simulink model "lab4_prep"  (R2023b)
settings: Solver=VariableStepAuto  StartTime=0.0  StopTime=10.0  RelTol=10e-10  AbsTol=10e-10
values from neighbouring files (symbols this model uses):
  Actrl = A + B*K - L*C    [lab4.m]
  Bctrl = [L, -B*K]    [lab4.m]
  C = [1 0 0 0; 0 0 1 0]    [lab4.m]
  Cctrl = K    [lab4.m]
  Dctrl = [zeros(1,2), -K]    [lab4.m]
  K = -place(A,B,p_K)    [lab4.m]
  Ulim = 5.875    [lab4.m]
  x0 = [0; 0; pi/24; 0]    [lab4.m]
settings Model: Creator=Darrian  LastModifiedBy=Darrian

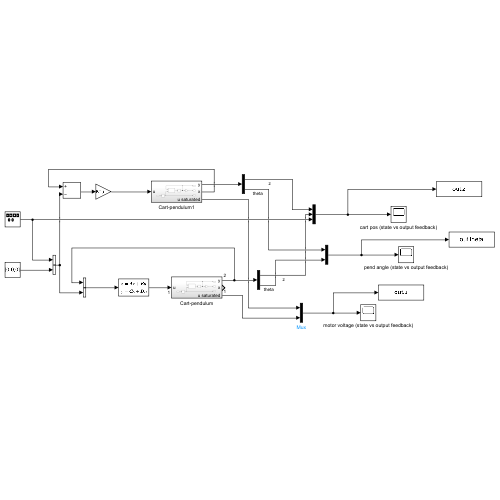
[thumbnail: Simulink's stored preview of the top-level diagram]
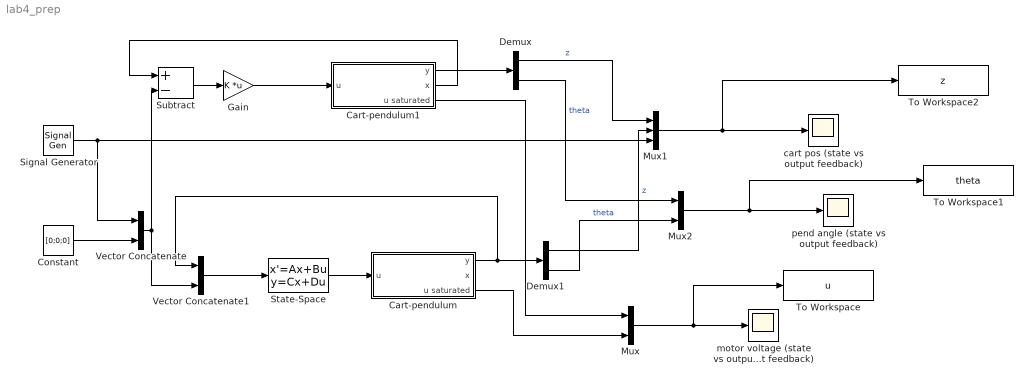
== system lab4_prep ==
  Cart-pendulum : Subsystem
  Cart-pendulum1 : Subsystem
  Constant : Constant  Value=[0;0;0]
  Demux : Demux  Outputs=2
  Demux1 : Demux  Outputs=2
  Gain : Gain  Gain=K  Multiplication=Matrix(K*u)
  Mux : Mux  Inputs=2
  Mux1 : Mux  Inputs=3
  Mux2 : Mux  Inputs=2
  Signal Generator : SignalGenerator  WaveForm=square  Amplitude=0.1  Frequency=0.1
  State-Space : StateSpace  A=Actrl  B=Bctrl  C=Cctrl  D=Dctrl  InitialCondition=0
  Subtract : Sum  Inputs=+-
  To Workspace : ToWorkspace  VariableName=u  SaveFormat=Timeseries  SampleTime=-1
  To Workspace1 : ToWorkspace  VariableName=theta  SaveFormat=Timeseries  SampleTime=-1
  To Workspace2 : ToWorkspace  VariableName=z  SaveFormat=Timeseries  SampleTime=-1
  Vector Concatenate : Concatenate
  Vector Concatenate1 : Concatenate
  cart pos (state vs output feedback) : Scope
  motor voltage (state vs output feedback) : Scope
  pend angle (state vs output feedback) : Scope
  wires:
  Gain/1 -> Cart-pendulum1/1(u)
  Constant/1 -> Vector Concatenate/2
  Signal Generator/1 -> Mux1/3, Vector Concatenate/1
  Subtract/1 -> Gain/1
  Cart-pendulum1/2(x) -> Subtract/1
  Cart-pendulum1/1(y) -> Demux/1
  State-Space/1 -> Cart-pendulum/1(u)
  Vector Concatenate/1 -> Subtract/2, Vector Concatenate1/2
  Vector Concatenate1/1 -> State-Space/1
  Cart-pendulum/1(y) -> Vector Concatenate1/1, Demux1/1
  Cart-pendulum1/3(u saturated) -> Mux/1
  Cart-pendulum/3(u saturated) -> Mux/2
  Demux/2 -> Mux2/1  "theta"
  Demux1/2 -> Mux2/2  "theta"
  Demux1/1 -> Mux1/2  "z"
  Demux/1 -> Mux1/1  "z"
  Mux/1 -> To Workspace/1, motor voltage (state vs output feedback)/1
  Mux1/1 -> To Workspace2/1, cart pos (state vs output feedback)/1
  Mux2/1 -> To Workspace1/1, pend angle (state vs output feedback)/1

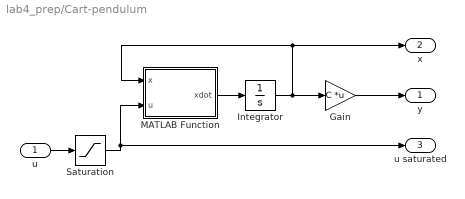
== system lab4_prep/Cart-pendulum ==
  u : Inport
  Gain : Gain  Gain=C  Multiplication=Matrix(K*u)
  Integrator : Integrator  InitialCondition=x0
  MATLAB Function : MATLAB Function  TreatAsAtomicUnit=on
  Saturation : Saturate  UpperLimit=Ulim  LowerLimit=-Ulim
  y : Outport
  x : Outport  Port=2
  u saturated : Outport  Port=3
  wires:
  u/1 -> Saturation/1
  Saturation/1 -> MATLAB Function/2(u), u saturated/1
  MATLAB Function/1(xdot) -> Integrator/1
  Integrator/1 -> Gain/1, x/1, MATLAB Function/1(x)
  Gain/1 -> y/1

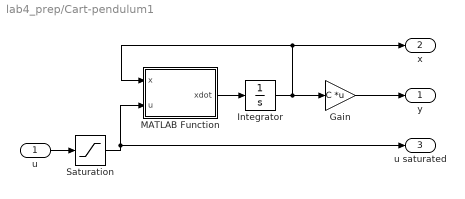
== system lab4_prep/Cart-pendulum1 ==
  u : Inport
  Gain : Gain  Gain=C  Multiplication=Matrix(K*u)
  Integrator : Integrator  InitialCondition=x0
  MATLAB Function : MATLAB Function  TreatAsAtomicUnit=on
  Saturation : Saturate  UpperLimit=Ulim  LowerLimit=-Ulim
  y : Outport
  x : Outport  Port=2
  u saturated : Outport  Port=3
  wires:
  u/1 -> Saturation/1
  Saturation/1 -> MATLAB Function/2(u), u saturated/1
  MATLAB Function/1(xdot) -> Integrator/1
  Integrator/1 -> Gain/1, x/1, MATLAB Function/1(x)
  Gain/1 -> y/1

== matlab function lab4_prep/Cart-pendulum/MATLAB Function ==
  data: x input; u input; xdot output
function xdot = cartpend(x,u)
xdot = cartpend(x,u);

== matlab function lab4_prep/Cart-pendulum1/MATLAB Function ==
  data: x input; u input; xdot output
function xdot = cartpend(x,u)
xdot = cartpend(x,u);
